simulink model "lafayettecopy"  (R2024a)
settings: Solver=VariableStepAuto  StartTime=0.0  StopTime=28  RelTol=1e-3
undefined symbols (not defined in the file): mass_vec, thrust_time_vec, thrust_vec, time_vec
libraries: slpidlib x3, aerolibanim x1, shared6dof x1
settings Model: Creator=amuss  LastModifiedBy=amuss

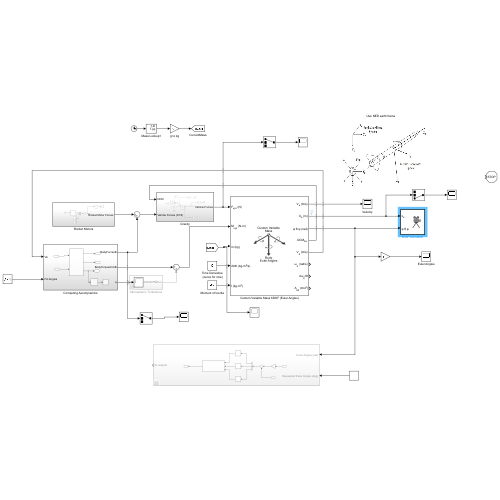
[thumbnail: Simulink's stored preview of the top-level diagram]
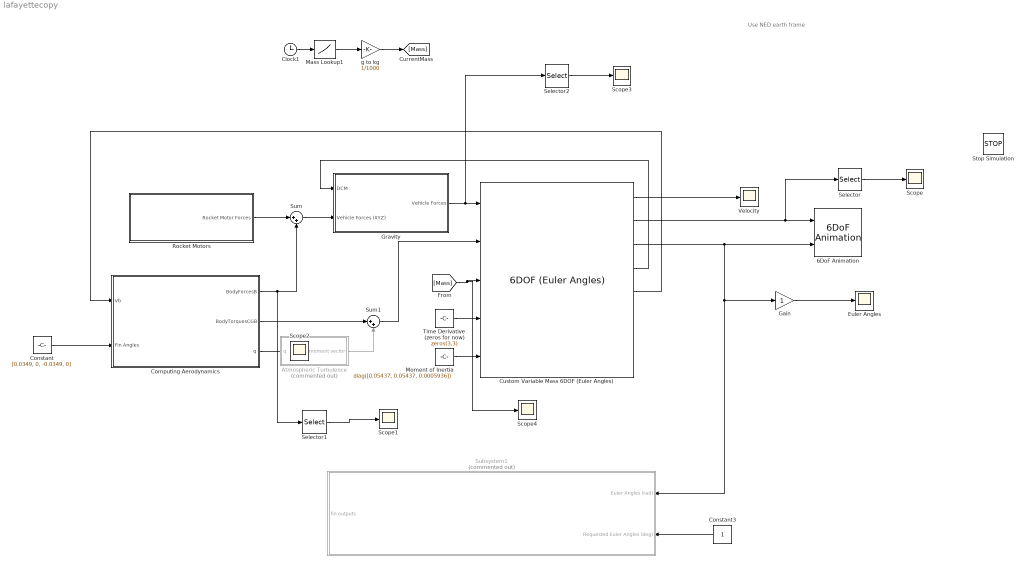
== system lafayettecopy ==
  note: Use NED earth frame
  6DoF Animation : aerolibanim/6DoF Animation  u1=[0 4000 -2000 2000 -5000 -3000]  u2=0.1  u3=250  u4=[4000 0 -5000]  u5=Fly alongside  u6=[2000 500 -3150]  u7=10  u8=on
  Atmospheric Turbulence : Subsystem  Commented=on
  Clock1 : Clock
  Computing Aerodynamics : Subsystem
  Constant : Constant  Value=[0.0349, 0, -0.0349, 0]
  Constant3 : Constant
  Custom Variable Mass 6DOF (Euler Angles) : shared6dof/6DOF (Euler Angles)  units=Metric (MKS)  mtype=Custom Variable  rep=Euler Angles  xme_0=[0 0 0]  Vm_0=[0 0 0]  eul_0=[0 0 0]  pm_0=[0 0 0]  mass_0=1.0  mass_e=0.5  mass_f=2.0  inertia=eye(3)  inertia_e=eye(3)  inertia_f=2*eye(3)  k_quat=1.0  vre_flag=off  abi_flag=off  aMode=0  xme_statename=''  Vm_statename=''  eul_statename=''  quat_statename=''  pm_statename=''  mass_statename=''
      settings: LibrarySourceBlock=aerolib6dof2/Custom Variable Mass 6DOF (Euler Angles)
  Euler Angles : Scope
  Gain : Gain
  Gravity : Subsystem
  Mass Lookup1 : Lookup_n-D  NumberOfTableDimensions=1  BreakpointsForDimension1=time_vec  Table=mass_vec  InternalRulePriority=Speed  RndMeth=Simplest
  Moment of Inertia : Constant  Value=diag([0.05437, 0.05437, 0.0005936])
  Rocket Motors : Subsystem
  Scope{,1..4} (5 alike) : Scope
  Selector : Selector  InputPortWidth=3  IndexOptions=Index vector (dialog)  Indices=[3]  OutputSizes=1
  Selector1 : Selector  InputPortWidth=3  IndexOptions=Index vector (dialog)  Indices=[1]  OutputSizes=1
  Selector2 : Selector  InputPortWidth=3  IndexOptions=Index vector (dialog)  Indices=[1]  OutputSizes=1
  Stop Simulation : Stop
  Subsystem1 : Subsystem  Commented=on
  Sum : Sum  Inputs=|++
  Sum1 : Sum  Inputs=|++
  Time Derivative (zeros for now) : Constant  Value=zeros(3,3)
  Velocity : Scope
  g to kg : Gain  Gain=1/1000
  wires:
  Computing Aerodynamics/1(BodyForcesB) -> Selector1/1, Sum/2
  Sum/1 -> Gravity/2(Vehicle Forces (XYZ))
  Moment of Inertia/1 -> Custom Variable Mass 6DOF (Euler Angles)/5
  Time Derivative (zeros for now)/1 -> Custom Variable Mass 6DOF (Euler Angles)/4
  Computing Aerodynamics/3(q) -> Scope2/1
  Atmospheric Turbulence/1(moment vector) -> Sum1/2
  Computing Aerodynamics/2(BodyTorquesCGB) -> Sum1/1
  Sum1/1 -> Custom Variable Mass 6DOF (Euler Angles)/2
  Custom Variable Mass 6DOF (Euler Angles)/1 -> Velocity/1
  Custom Variable Mass 6DOF (Euler Angles)/3 -> Subsystem1/1(Euler Angles (rad)), Gain/1, 6DoF Animation/2
  Gain/1 -> Euler Angles/1
  Constant3/1 -> Subsystem1/2(Requested Euler Angles (deg))
  Custom Variable Mass 6DOF (Euler Angles)/4 -> Gravity/1(DCM)
  Custom Variable Mass 6DOF (Euler Angles)/5 -> Computing Aerodynamics/1(Vb)
  Clock1/1 -> Mass Lookup1/1
  [Mass] -> Scope4/1, Custom Variable Mass 6DOF (Euler Angles)/3
  Constant/1 -> Computing Aerodynamics/2(Fin Angles)
  Rocket Motors/1(Rocket Motor Forces) -> Sum/1
  Gravity/1(Vehicle Forces) -> Selector2/1, Custom Variable Mass 6DOF (Euler Angles)/1
  Custom Variable Mass 6DOF (Euler Angles)/2 -> Selector/1, 6DoF Animation/1
  Selector/1 -> Scope/1
  Selector1/1 -> Scope1/1
  Selector2/1 -> Scope3/1
  Mass Lookup1/1 -> g to kg/1
  g to kg/1 -> [Mass]

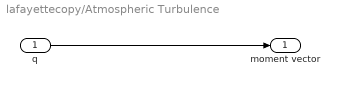
== system lafayettecopy/Atmospheric Turbulence ==
  q : Inport
  moment vector : Outport
  wires:
  q/1 -> moment vector/1

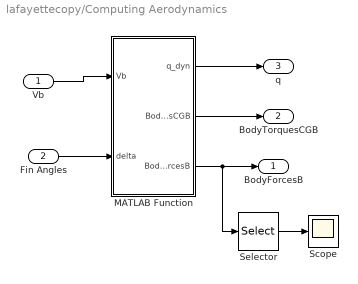
== system lafayettecopy/Computing Aerodynamics ==
  Vb : Inport
  Fin Angles : Inport  Port=2
  MATLAB Function : MATLAB Function  TreatAsAtomicUnit=on
  Scope : Scope
  Selector : Selector  InputPortWidth=3  IndexOptions=Index vector (dialog)  Indices=[1]  OutputSizes=1
  BodyForcesB : Outport
  BodyTorquesCGB : Outport  Port=2
  q : Outport  Port=3
  wires:
  Vb/1 -> MATLAB Function/1(Vb)
  Fin Angles/1 -> MATLAB Function/2(delta)
  MATLAB Function/1(q_dyn) -> q/1
  MATLAB Function/2(BodyTorquesCGB) -> BodyTorquesCGB/1
  MATLAB Function/3(BodyForcesB) -> Selector/1, BodyForcesB/1
  Selector/1 -> Scope/1

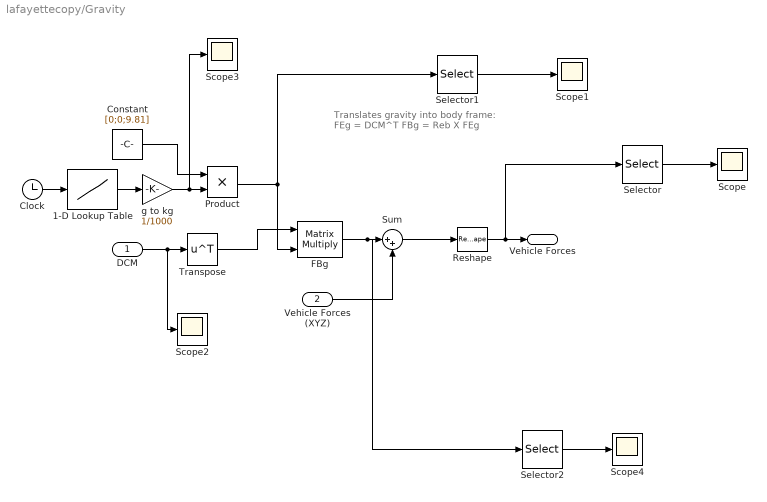
== system lafayettecopy/Gravity ==
  note: Translates gravity into body frame:
      | FEg = DCM^T
      | FBg = Reb X FEg
  DCM : Inport
  Vehicle Forces (XYZ) : Inport  Port=2
  1-D Lookup Table : Lookup_n-D  NumberOfTableDimensions=1  BreakpointsForDimension1=time_vec  Table=mass_vec  InternalRulePriority=Speed  RndMeth=Simplest
  Clock : Clock
  Constant : Constant  Value=[0;0;9.81]  VectorParams1D=off
  FBg : Product  Multiplication=Matrix(*)
  Product : Product
  Reshape : Reshape
  Scope{,1..4} (5 alike) : Scope
  Selector : Selector  InputPortWidth=3  IndexOptions=Index vector (dialog)  Indices=[1]  OutputSizes=1
  Selector1 : Selector  InputPortWidth=3  IndexOptions=Index vector (dialog)  Indices=[3]  OutputSizes=1
  Selector2 : Selector  InputPortWidth=3  IndexOptions=Index vector (dialog)  Indices=[1]  OutputSizes=1
  Sum : Sum  Inputs=|++
  Transpose : Math  Operator=transpose
  g to kg : Gain  Gain=1/1000
  Vehicle Forces : Outport
  wires:
  DCM/1 -> Scope2/1, Transpose/1
  Vehicle Forces (XYZ)/1 -> Sum/2
  Sum/1 -> Reshape/1
  1-D Lookup Table/1 -> g to kg/1
  FBg/1 -> Selector2/1, Sum/1
  Reshape/1 -> Selector/1, Vehicle Forces/1
  Constant/1 -> Product/1
  Transpose/1 -> FBg/1
  Product/1 -> FBg/2, Selector1/1
  Selector/1 -> Scope/1
  Selector1/1 -> Scope1/1
  Clock/1 -> 1-D Lookup Table/1
  g to kg/1 -> Scope3/1, Product/2
  Selector2/1 -> Scope4/1

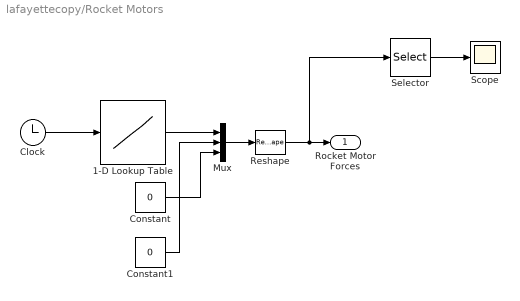
== system lafayettecopy/Rocket Motors ==
  1-D Lookup Table : Lookup_n-D  NumberOfTableDimensions=1  BreakpointsForDimension1=thrust_time_vec  Table=thrust_vec  InternalRulePriority=Speed  RndMeth=Simplest
  Clock : Clock
  Constant : Constant  Value=0
  Constant1 : Constant  Value=0
  Mux : Mux  Inputs=3
  Reshape : Reshape  OutputDimensionality=Customize  OutputDimensions=[3,1]
  Scope : Scope
  Selector : Selector  InputPortWidth=3  IndexOptions=Index vector (dialog)  Indices=[1]  OutputSizes=1
  Rocket Motor Forces : Outport
  wires:
  Clock/1 -> 1-D Lookup Table/1
  1-D Lookup Table/1 -> Mux/1
  Constant/1 -> Mux/3
  Constant1/1 -> Mux/2
  Mux/1 -> Reshape/1
  Reshape/1 -> Selector/1, Rocket Motor Forces/1
  Selector/1 -> Scope/1

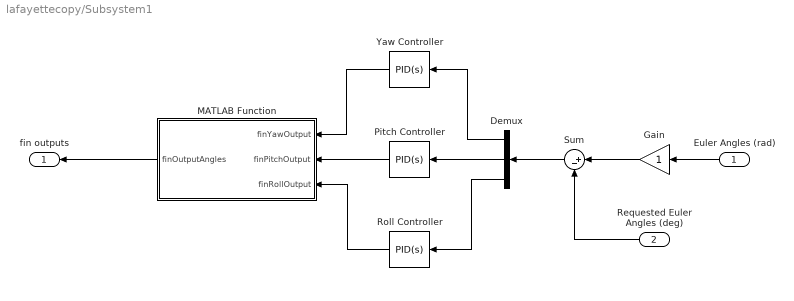
== system lafayettecopy/Subsystem1 ==
  Euler Angles (rad) : Inport
  Requested Euler Angles (deg) : Inport  Port=2
  Demux : Demux  Outputs=3
  Gain : Gain
  MATLAB Function : MATLAB Function  TreatAsAtomicUnit=on
  Pitch Controller : slpidlib/PID Controller  Controller=PID  Form=Parallel  TimeDomain=Continuous-time  UseExternalTs=off  SampleTime=-1  IntegratorMethod=Forward Euler  FilterMethod=Forward Euler  ControllerParametersSource=internal  P=1  I=1  UseKiTs=off  D=0  UseExternalDerivativeSource=off  N=100  UseFilter=on  TunerSelectOption=Transfer Function Based (PID Tuner App)  InitialConditionSource=internal  InitialConditionForIntegrator=0  InitialConditionForFilter=0  DifferentiatorICPrevScaledInput=0  ExternalReset=none  TrackingMode=off  Kt=1  LimitOutput=off  SatLimitsSource=internal  UpperSaturationLimit=inf  LowerSaturationLimit=-inf  LinearizeAsGain=on  AntiWindupMode=none  Kb=1  LimitIntegrator=off  UpperIntegratorSaturationLimit=inf  LowerIntegratorSaturationLimit=-inf  POutMin=[]  POutMax=[]  IOutMin=[]  IOutMax=[]  DOutMin=[]  DOutMax=[]  NOutMin=[]  NOutMax=[]  SumOutMin=[]  SumOutMax=[]  SaturationOutMin=[]  SaturationOutMax=[]  PParamMin=[]  PParamMax=[]  IParamMin=[]  IParamMax=[]  DParamMin=[]  DParamMax=[]  NParamMin=[]  NParamMax=[]  KbParamMin=[]  KbParamMax=[]  KtParamMin=[]  KtParamMax=[]  KbOutMin=[]  KbOutMax=[]  KtOutMin=[]  KtOutMax=[]  IntegratorOutMin=[]  IntegratorOutMax=[]  FilterOutMin=[]  FilterOutMax=[]  SumI1OutMin=[]  SumI1OutMax=[]  SumI2OutMin=[]  SumI2OutMax=[]  SumI3OutMin=[]  SumI3OutMax=[]  SumI4OutMin=[]  SumI4OutMax=[]  SumDOutMin=[]  SumDOutMax=[]  DifferentiatorOutMin=[]  DifferentiatorOutMax=[]  FilterDiffOutCoefMin=[]  FilterDiffOutCoefMax=[]  ReciprocalOutMin=[]  ReciprocalOutMax=[]  SumDenOutMin=[]  SumDenOutMax=[]  SumNumOutMin=[]  SumNumOutMax=[]  DivideOutMin=[]  DivideOutMax=[]  UdiffTsProdOutMin=[]  UdiffTsProdOutMax=[]  NTsProdOutMin=[]  NTsProdOutMax=[]  UintegralTsProdOutMin=[]  UintegralTsProdOutMax=[]  UngainTsProdOutMin=[]  UngainTsProdOutMax=[]  ClampingZeroOutDataTypeStr=Inherit: Inherit via back propagation  ClampingZeroOutMin=[]  ClampingZeroOutMax=[]  FilterDenConstantOutDataTypeStr=Inherit: Inherit via back propagation  FilterDenConstantOutMin=[]  FilterDenConstantOutMax=[]  PCopyOutDataTypeStr=Inherit: Inherit via back propagation  PCopyOutMin=[]  PCopyOutMax=[]  NCopyOutDataTypeStr=Inherit: Inherit via back propagation  NCopyOutMin=[]  NCopyOutMax=[]  IntegratorContinuousStateAttributes=''  IntegratorStateMustResolveToSignalObject=off  IntegratorRTWStateStorageClass=Auto  FilterContinuousStateAttributes=''  FilterStateMustResolveToSignalObject=off  FilterRTWStateStorageClass=Auto  ParallelPVariant=InternalParameters  IdealPVariant=Disabled  IVariant=InternalParameters  DVariant=InternalParameters  IntegratorVariant=Continuous  SatVariant=Disabled  AWVariant=Passthrough  PCopyVariant=Disabled  TRVariant=Disabled  FdbkBlocksVariant=Forward  IdealPFdbkVariant=Disabled  SatFdbkVariant=Disabled  DerivativeFilterVariant=ContFilter  NVariant=InternalParameters  NCopyVariant=Disabled  FilterICVariant=InternalICsFilter  IntegratorICVariant=InternalICs  ExternalResetVariant=Disabled  TRSumVariant=Passthrough  SumFdbkVariant=Disabled  SumVariant=Sum_PID  TsampFilterVariant=InternalTs  TsampNgainVariant=Passthrough  TsampIntegralVariant=Disabled_SignalSpec  ExternalSaturationOutDataTypeStr=Inherit: Same as second input  DerivativeSourceVariant=ErrorSignal
  Roll Controller : slpidlib/PID Controller  Controller=PID  Form=Parallel  TimeDomain=Continuous-time  UseExternalTs=off  SampleTime=-1  IntegratorMethod=Forward Euler  FilterMethod=Forward Euler  ControllerParametersSource=internal  P=1  I=1  UseKiTs=off  D=0  UseExternalDerivativeSource=off  N=100  UseFilter=on  TunerSelectOption=Transfer Function Based (PID Tuner App)  InitialConditionSource=internal  InitialConditionForIntegrator=0  InitialConditionForFilter=0  DifferentiatorICPrevScaledInput=0  ExternalReset=none  TrackingMode=off  Kt=1  LimitOutput=off  SatLimitsSource=internal  UpperSaturationLimit=inf  LowerSaturationLimit=-inf  LinearizeAsGain=on  AntiWindupMode=none  Kb=1  LimitIntegrator=off  UpperIntegratorSaturationLimit=inf  LowerIntegratorSaturationLimit=-inf  POutMin=[]  POutMax=[]  IOutMin=[]  IOutMax=[]  DOutMin=[]  DOutMax=[]  NOutMin=[]  NOutMax=[]  SumOutMin=[]  SumOutMax=[]  SaturationOutMin=[]  SaturationOutMax=[]  PParamMin=[]  PParamMax=[]  IParamMin=[]  IParamMax=[]  DParamMin=[]  DParamMax=[]  NParamMin=[]  NParamMax=[]  KbParamMin=[]  KbParamMax=[]  KtParamMin=[]  KtParamMax=[]  KbOutMin=[]  KbOutMax=[]  KtOutMin=[]  KtOutMax=[]  IntegratorOutMin=[]  IntegratorOutMax=[]  FilterOutMin=[]  FilterOutMax=[]  SumI1OutMin=[]  SumI1OutMax=[]  SumI2OutMin=[]  SumI2OutMax=[]  SumI3OutMin=[]  SumI3OutMax=[]  SumI4OutMin=[]  SumI4OutMax=[]  SumDOutMin=[]  SumDOutMax=[]  DifferentiatorOutMin=[]  DifferentiatorOutMax=[]  FilterDiffOutCoefMin=[]  FilterDiffOutCoefMax=[]  ReciprocalOutMin=[]  ReciprocalOutMax=[]  SumDenOutMin=[]  SumDenOutMax=[]  SumNumOutMin=[]  SumNumOutMax=[]  DivideOutMin=[]  DivideOutMax=[]  UdiffTsProdOutMin=[]  UdiffTsProdOutMax=[]  NTsProdOutMin=[]  NTsProdOutMax=[]  UintegralTsProdOutMin=[]  UintegralTsProdOutMax=[]  UngainTsProdOutMin=[]  UngainTsProdOutMax=[]  ClampingZeroOutDataTypeStr=Inherit: Inherit via back propagation  ClampingZeroOutMin=[]  ClampingZeroOutMax=[]  FilterDenConstantOutDataTypeStr=Inherit: Inherit via back propagation  FilterDenConstantOutMin=[]  FilterDenConstantOutMax=[]  PCopyOutDataTypeStr=Inherit: Inherit via back propagation  PCopyOutMin=[]  PCopyOutMax=[]  NCopyOutDataTypeStr=Inherit: Inherit via back propagation  NCopyOutMin=[]  NCopyOutMax=[]  IntegratorContinuousStateAttributes=''  IntegratorStateMustResolveToSignalObject=off  IntegratorRTWStateStorageClass=Auto  FilterContinuousStateAttributes=''  FilterStateMustResolveToSignalObject=off  FilterRTWStateStorageClass=Auto  ParallelPVariant=InternalParameters  IdealPVariant=Disabled  IVariant=InternalParameters  DVariant=InternalParameters  IntegratorVariant=Continuous  SatVariant=Disabled  AWVariant=Passthrough  PCopyVariant=Disabled  TRVariant=Disabled  FdbkBlocksVariant=Forward  IdealPFdbkVariant=Disabled  SatFdbkVariant=Disabled  DerivativeFilterVariant=ContFilter  NVariant=InternalParameters  NCopyVariant=Disabled  FilterICVariant=InternalICsFilter  IntegratorICVariant=InternalICs  ExternalResetVariant=Disabled  TRSumVariant=Passthrough  SumFdbkVariant=Disabled  SumVariant=Sum_PID  TsampFilterVariant=InternalTs  TsampNgainVariant=Passthrough  TsampIntegralVariant=Disabled_SignalSpec  ExternalSaturationOutDataTypeStr=Inherit: Same as second input  DerivativeSourceVariant=ErrorSignal
  Sum : Sum  Inputs=|+-
  Yaw Controller : slpidlib/PID Controller  Controller=PID  Form=Parallel  TimeDomain=Continuous-time  UseExternalTs=off  SampleTime=-1  IntegratorMethod=Forward Euler  FilterMethod=Forward Euler  ControllerParametersSource=internal  P=1  I=1  UseKiTs=off  D=0  UseExternalDerivativeSource=off  N=100  UseFilter=on  TunerSelectOption=Transfer Function Based (PID Tuner App)  InitialConditionSource=internal  InitialConditionForIntegrator=0  InitialConditionForFilter=0  DifferentiatorICPrevScaledInput=0  ExternalReset=none  TrackingMode=off  Kt=1  LimitOutput=off  SatLimitsSource=internal  UpperSaturationLimit=inf  LowerSaturationLimit=-inf  LinearizeAsGain=on  AntiWindupMode=none  Kb=1  LimitIntegrator=off  UpperIntegratorSaturationLimit=inf  LowerIntegratorSaturationLimit=-inf  POutMin=[]  POutMax=[]  IOutMin=[]  IOutMax=[]  DOutMin=[]  DOutMax=[]  NOutMin=[]  NOutMax=[]  SumOutMin=[]  SumOutMax=[]  SaturationOutMin=[]  SaturationOutMax=[]  PParamMin=[]  PParamMax=[]  IParamMin=[]  IParamMax=[]  DParamMin=[]  DParamMax=[]  NParamMin=[]  NParamMax=[]  KbParamMin=[]  KbParamMax=[]  KtParamMin=[]  KtParamMax=[]  KbOutMin=[]  KbOutMax=[]  KtOutMin=[]  KtOutMax=[]  IntegratorOutMin=[]  IntegratorOutMax=[]  FilterOutMin=[]  FilterOutMax=[]  SumI1OutMin=[]  SumI1OutMax=[]  SumI2OutMin=[]  SumI2OutMax=[]  SumI3OutMin=[]  SumI3OutMax=[]  SumI4OutMin=[]  SumI4OutMax=[]  SumDOutMin=[]  SumDOutMax=[]  DifferentiatorOutMin=[]  DifferentiatorOutMax=[]  FilterDiffOutCoefMin=[]  FilterDiffOutCoefMax=[]  ReciprocalOutMin=[]  ReciprocalOutMax=[]  SumDenOutMin=[]  SumDenOutMax=[]  SumNumOutMin=[]  SumNumOutMax=[]  DivideOutMin=[]  DivideOutMax=[]  UdiffTsProdOutMin=[]  UdiffTsProdOutMax=[]  NTsProdOutMin=[]  NTsProdOutMax=[]  UintegralTsProdOutMin=[]  UintegralTsProdOutMax=[]  UngainTsProdOutMin=[]  UngainTsProdOutMax=[]  ClampingZeroOutDataTypeStr=Inherit: Inherit via back propagation  ClampingZeroOutMin=[]  ClampingZeroOutMax=[]  FilterDenConstantOutDataTypeStr=Inherit: Inherit via back propagation  FilterDenConstantOutMin=[]  FilterDenConstantOutMax=[]  PCopyOutDataTypeStr=Inherit: Inherit via back propagation  PCopyOutMin=[]  PCopyOutMax=[]  NCopyOutDataTypeStr=Inherit: Inherit via back propagation  NCopyOutMin=[]  NCopyOutMax=[]  IntegratorContinuousStateAttributes=''  IntegratorStateMustResolveToSignalObject=off  IntegratorRTWStateStorageClass=Auto  FilterContinuousStateAttributes=''  FilterStateMustResolveToSignalObject=off  FilterRTWStateStorageClass=Auto  ParallelPVariant=InternalParameters  IdealPVariant=Disabled  IVariant=InternalParameters  DVariant=InternalParameters  IntegratorVariant=Continuous  SatVariant=Disabled  AWVariant=Passthrough  PCopyVariant=Disabled  TRVariant=Disabled  FdbkBlocksVariant=Forward  IdealPFdbkVariant=Disabled  SatFdbkVariant=Disabled  DerivativeFilterVariant=ContFilter  NVariant=InternalParameters  NCopyVariant=Disabled  FilterICVariant=InternalICsFilter  IntegratorICVariant=InternalICs  ExternalResetVariant=Disabled  TRSumVariant=Passthrough  SumFdbkVariant=Disabled  SumVariant=Sum_PID  TsampFilterVariant=InternalTs  TsampNgainVariant=Passthrough  TsampIntegralVariant=Disabled_SignalSpec  ExternalSaturationOutDataTypeStr=Inherit: Same as second input  DerivativeSourceVariant=ErrorSignal
  fin outputs : Outport
  wires:
  Euler Angles (rad)/1 -> Gain/1
  Requested Euler Angles (deg)/1 -> Sum/2
  Gain/1 -> Sum/1
  Sum/1 -> Demux/1
  Demux/1 -> Yaw Controller/1
  Demux/2 -> Pitch Controller/1
  Demux/3 -> Roll Controller/1
  Yaw Controller/1 -> MATLAB Function/1(finYawOutput)
  Pitch Controller/1 -> MATLAB Function/2(finPitchOutput)
  Roll Controller/1 -> MATLAB Function/3(finRollOutput)
  MATLAB Function/1(finOutputAngles) -> fin outputs/1

== matlab function lafayettecopy/Computing Aerodynamics/MATLAB Function ==
  data: Vb input; q_dyn output; delta input; BodyTorquesCGB output; BodyForcesB output
function [q_dyn, BodyTorquesCGB, BodyForcesB] = finAero(Vb, delta)
% delta = [d1; d2; d3; d4] in radians, fins at 0,90,180,270 deg (X-config)
% Note: this seems right intuitively. Stems from rxF for all four fins.
% May need to tune Cl, l, R, Sf. Also may need to add induced drag for
% higher fidelity.

% --- parameters ---
rho   = 1.225;          % kg/m^3
Sf    = 0.0008;         % single-fin planform area [m^2]
CLd   = 3.0;            % lift slope per rad (tune/estimate)
l     = 0.35;           % axial arm CG->fin AC [m]
R     = 0.04;           % radial arm (body radius to fin AC) [m]
CD0   = 0.6;            % baseline drag coeff (optional)
Sref  = pi*R^2;         % ref frontal area

% --- dynamics ---
Vmag = norm(Vb);
q_dyn = 0.5*rho*Vmag*Vmag;
k   = q_dyn * Sf * CLd;
kl  = k * l;
kR  = k * R;
vhat = Vb / (Vmag + 1e-6);

d1=delta(1); d2=delta(2); d3=delta(3); d4=delta(4);

% Drag force
Drag = -q_dyn*Sref*CD0*vhat;           % baseline body drag (optional)
Dragx = Drag(1); Dragy = Drag(2); Dragz = Drag(3);

% Body Forces
Fx = Dragx;
Fy =  k*( d1 - d3) + Dragy;
Fz =  k*(-d2 + d4) + Dragz;
BodyForcesB  = [Fx; Fy; Fz];

% Moments about CG in body frame
Mx = -kR*(d1 + d2 + d3 + d4);
My =  kl*(d2 - d4);
Mz =  kl*(d1 - d3);
BodyTorquesCGB = [Mx; My; Mz];
end

== matlab function lafayettecopy/Subsystem1/MATLAB Function ==
  data: finYawOutput input; finOutputAngles output; finPitchOutput input; finRollOutput input
function finOutputAngles = fcn(finYawOutput,finPitchOutput,finRollOutput)

y = u;
